simulink model "Rail_MonMeUn"  (R2016b)
settings: configuration reference "CodeGenConfigSet" (kept outside this file)
values from neighbouring files (symbols this model uses):
  Rail_dvolMeUnMonSetMin_C = Calibration.Parameter    [init_Rail_MonMeUn.m]
  Rail_dvolMeUnOvrRun_CUR = Calibration.Parameter    [init_Rail_MonMeUn.m]
  Rail_dvolMeUnOvrRun_CURX = Calibration.Parameter    [init_Rail_MonMeUn.m]
  Rail_dvolMonHPUnTolc_CUR = Calibration.Parameter    [init_Rail_MonMeUn.m]
  Rail_dvolMonHPUnTolc_CURX = Calibration.Parameter    [init_Rail_MonMeUn.m]
  Rail_dvolMonIdlMax_C = Calibration.Parameter    [init_Rail_MonMeUn.m]
  Rail_dvolMonLeakTolc_CUR = Calibration.Parameter    [init_Rail_MonMeUn.m]
  Rail_dvolMonLeakTolc_CURX = Calibration.Parameter    [init_Rail_MonMeUn.m]
  Rail_nMonIdlMax_C = Calibration.Parameter    [init_Rail_MonMeUn.m]
  Rail_pMeUnDvtMax_CUR = Calibration.Parameter    [init_Rail_MonMeUn.m]
  Rail_pMeUnDvtMax_CURX = Calibration.Parameter    [init_Rail_MonMeUn.m]
  Rail_pMeUnDvtMin2_CUR = Calibration.Parameter    [init_Rail_MonMeUn.m]
  Rail_pMeUnDvtMin2_CURX = Calibration.Parameter    [init_Rail_MonMeUn.m]
  Rail_pMeUnDvtMin_CUR = Calibration.Parameter    [init_Rail_MonMeUn.m]
  Rail_pMeUnDvtMin_CURX = Calibration.Parameter    [init_Rail_MonMeUn.m]
  Rail_pMeUnFltMin_CUR = Calibration.Parameter    [init_Rail_MonMeUn.m]
  Rail_pMeUnFltMin_CURX = Calibration.Parameter    [init_Rail_MonMeUn.m]
  Rail_pMeUnMonFltMax2_C = Calibration.Parameter    [init_Rail_MonMeUn.m]
  Rail_pMeUnMonFltMax_C = Calibration.Parameter    [init_Rail_MonMeUn.m]
  Rail_pMonDvtMax_C = Calibration.Parameter    [init_Rail_MonMeUn.m]
  Rail_qMeUnMonLoIdl_C = Calibration.Parameter    [init_Rail_MonMeUn.m]
  Rail_qMonUnBalMax_C = Calibration.Parameter    [init_Rail_MonMeUn.m]
  Rail_stMeUnMonRls_C = Calibration.Parameter    [init_Rail_MonMeUn.m]
  Rail_tiMeUn0Deb_C = Calibration.Parameter    [init_Rail_MonMeUn.m]
  Rail_tiMeUn10Deb_C = Calibration.Parameter    [init_Rail_MonMeUn.m]
  Rail_tiMeUn22Deb_C = Calibration.Parameter    [init_Rail_MonMeUn.m]
  Rail_tiMeUn2Deb_C = Calibration.Parameter    [init_Rail_MonMeUn.m]
  Rail_tiMeUn3Deb_C = Calibration.Parameter    [init_Rail_MonMeUn.m]
  Rail_tiMeUn42Deb_C = Calibration.Parameter    [init_Rail_MonMeUn.m]
  Rail_tiMeUn4Deb_C = Calibration.Parameter    [init_Rail_MonMeUn.m]
  Rail_tiMeUn7Deb_C = Calibration.Parameter    [init_Rail_MonMeUn.m]
  Rail_tiMeUn8Deb_C = Calibration.Parameter    [init_Rail_MonMeUn.m]
  Rail_tMeUnMonLoIdl_C = Calibration.Parameter    [init_Rail_MonMeUn.m]
undefined symbols (not defined in the file or in its folder): Rail_MonMeUn_DT, RailCtl_State_conv
libraries: CXLib x27, simulink x18
settings Model: Creator=lenovo  LastModifiedBy=liutao
settings ConfigSetRef: SourceLocation=Base Workspace

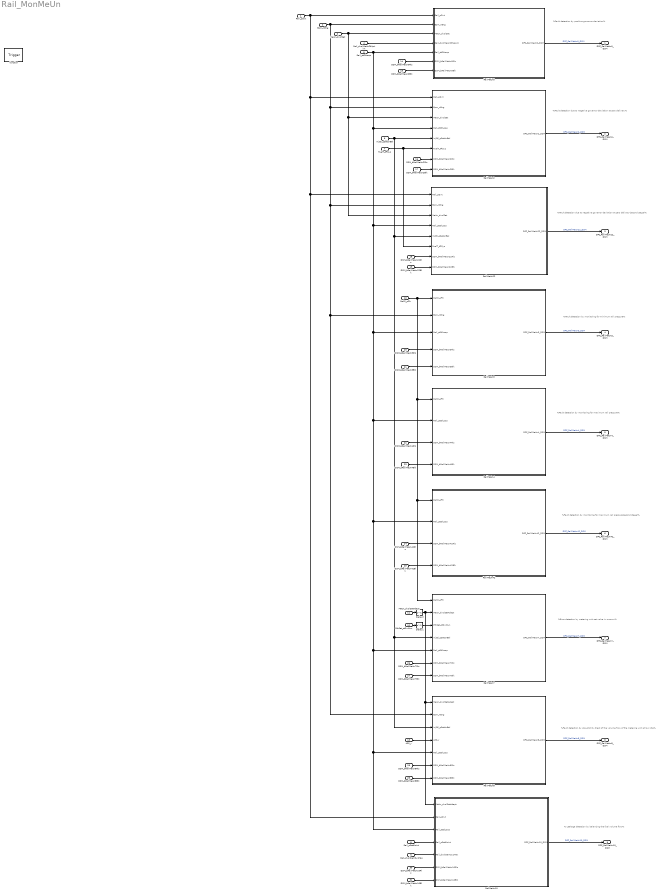
== system Rail_MonMeUn ==
  note: % Leakage detection by balancing the fuel volume flow%
  note: %Fault detection by plausibility check of the volume flow of the metering unit at low idle%
  note: %Error detection by metering unit set value in overrun%
  note: %Fault detection by monitoring for maximum rail pressure(second stage)%
  note: %Fault detection by monitoring for maximum rail pressure%
  note: %Fault detection by monitoring for minimum rail pressure%
  note: %Fault detection due to negative governor deviation at zero delivery(second stage)%
  note: %Fault detection due to negative governor deviation at zero delivery%
  note: %Fault detection by positive governor deviation%
  Rail_pDvt : Inport  Tag=bar  Description=Governor deviation of the rail pressure governor  OutMin=-2500  OutMax=2500  OutDataTypeStr=RailPressure_bar
  Epm_nEng : Inport  Tag=rpm  Description=Engine speed  Port=2  OutMin=0  OutMax=6000  OutDataTypeStr=EngSpeed_rpm
  MeUn_dvolSet : Inport  Tag=mm^3/s  Description=Setpoint value (volume flow) of rail pressure governing  Port=3  OutMin=-327670  OutMax=327670  OutDataTypeStr=FuelVol_mm3_s
  Rail_dvolMeUnCtlUpLim : Inport  Tag=mm^3/s  Description=Upper actuator value limit for pressure governing by metering unit  Port=4  OutMin=0  OutMax=327670  OutDataTypeStr=FuelVol_mm3_s
  Rail_stCtlLoop : Inport  Description=State of the rail pressure governor control  Port=5  OutDataTypeStr=Enum: RailCtl_State_conv
  InjCtl_qSetUnBal : Inport  Tag=mg/hub  Description=Current injection quantity  Port=6  OutMin=-319  OutMax=319  OutDataTypeStr=FuelMass_mg_hub
  FuelT_tFlSys : Inport  Tag=deg  Description=Fuel system temperature  Port=7  OutMin=-50  OutMax=200  OutDataTypeStr=Temp_deg
  Rail_pSetPoint : Inport  Tag=bar  Description=Rail pressure setpoint  Port=8  OutMin=-2500  OutMax=2500  OutDataTypeStr=RailPressure_bar
  Rail_dvolDemSysMax : Inport  Tag=mm^3/s  Description=Volume flow requested overall for a maximum tolerated injection system  Port=9  OutMin=-327680  OutMax=327670  OutDataTypeStr=FuelVol_mm3_s
  RailP_pFlt : Inport  Tag=bar  Description=Maximum rail pressure of the last 10 sampling cycle  Port=10  OutMin=0  OutMax=2500  OutDataTypeStr=RailPressure_bar
  MeUn_dvolSetAdapt : Inport  Tag=mm^3/s  Description=Correction value of the adaption of the metering unit  Port=11  OutMin=-327680  OutMax=327670  OutDataTypeStr=FuelVol_mm3_s
  PthSet_stOvrRun : Inport  Description=State of overrun detection (0: No overrun; 1: overrun)  Port=12  OutMin=0  OutMax=1  OutDataTypeStr=boolean
  APP_r : Inport  Tag=%  Description=Acceleration pedal sensor 1 value after fault handling  Port=13  OutMin=0  OutMax=100  OutDataTypeStr=Accpedal_rate
  DSM_bRailMeUn0Rls : Inport  Description=state of FId_RailMeUn0Rls  Port=14  OutMin=0  OutMax=1  OutDataTypeStr=boolean
  DSM_bRailMeUn0Blk : Inport  Description=state of FId_RailMeUn0Blk  Port=15  OutMin=0  OutMax=1  OutDataTypeStr=boolean
  DSM_bRailMeUn2Rls : Inport  Description=state of FId_RailMeUn2Rls  Port=16  OutMin=0  OutMax=1  OutDataTypeStr=boolean
  DSM_bRailMeUn2Blk : Inport  Description=state of FId_RailMeUn2Blk  Port=17  OutMin=0  OutMax=1  OutDataTypeStr=boolean
  DSM_bRailMeUn22Rls : Inport  Description=state of FId_RailMeUn22Rls  Port=18  OutMin=0  OutMax=1  OutDataTypeStr=boolean
  DSM_bRailMeUn22Blk : Inport  Description=state of FId_RailMeUn22Blk  Port=19  OutMin=0  OutMax=1  OutDataTypeStr=boolean
  DSM_bRailMeUn3Rls : Inport  Description=state of FId_RailMeUn3Rls  Port=20  OutMin=0  OutMax=1  OutDataTypeStr=boolean
  DSM_bRailMeUn3Blk : Inport  Description=state of FId_RailMeUn3Blk  Port=21  OutMin=0  OutMax=1  OutDataTypeStr=boolean
  DSM_bRailMeUn4Rls : Inport  Description=state of FId_RailMeUn4Rls  Port=22  OutMin=0  OutMax=1  OutDataTypeStr=boolean
  DSM_bRailMeUn4Blk : Inport  Description=state of FId_RailMeUn4Blk  Port=23  OutMin=0  OutMax=1  OutDataTypeStr=boolean
  DSM_bRailMeUn42Rls : Inport  Description=state of FId_RailMeUn42Rls  Port=24  OutMin=0  OutMax=1  OutDataTypeStr=boolean
  DSM_bRailMeUn42Blk : Inport  Description=state of FId_RailMeUn42Blk  Port=25  OutMin=0  OutMax=1  OutDataTypeStr=boolean
  DSM_bRailMeUn7Rls : Inport  Description=state of FId_RailMeUn7Rls  Port=26  OutMin=0  OutMax=1  OutDataTypeStr=boolean
  DSM_bRailMeUn7Blk : Inport  Description=state of FId_RailMeUn7Blk  Port=27  OutMin=0  OutMax=1  OutDataTypeStr=boolean
  DSM_bRailMeUn8Rls : Inport  Description=state of FId_RailMeUn8Rls  Port=28  OutMin=0  OutMax=1  OutDataTypeStr=boolean
  DSM_bRailMeUn8Blk : Inport  Description=state of FId_RailMeUn8Blk  Port=29  OutMin=0  OutMax=1  OutDataTypeStr=boolean
  DSM_bRailMeUn10Rls : Inport  Description=state of FId_RailMeUn10Rls  Port=30  OutMin=0  OutMax=1  OutDataTypeStr=boolean
  DSM_bRailMeUn10Blk : Inport  Description=state of FId_RailMeUn10Blk  Port=31  OutMin=0  OutMax=1  OutDataTypeStr=boolean
  function : TriggerPort  TriggerType=function-call  VariantControl=Variant
  Delay1 : Delay  DelayLength=1  InitialCondition=0
  Delay2 : Delay  DelayLength=1  InitialCondition=0
  RailMeUn0 : Subsystem
  RailMeUn10 : Subsystem
  RailMeUn2 : Subsystem
  RailMeUn22 : Subsystem
  RailMeUn3 : Subsystem
  RailMeUn4 : Subsystem
  RailMeUn42 : Subsystem
  RailMeUn7 : Subsystem
  RailMeUn8 : Subsystem
  DFC_RailMeUn0_DSM : Outport  Description=state of DFC_RailMeUn0  OutMin=0  OutMax=1  OutDataTypeStr=boolean
  DFC_RailMeUn2_DSM : Outport  Description=state of DFC_RailMeUn2  Port=2  OutMin=0  OutMax=1  OutDataTypeStr=boolean
  DFC_RailMeUn22_DSM : Outport  Description=state of DFC_RailMeUn22  Port=3  OutMin=0  OutMax=1  OutDataTypeStr=boolean
  DFC_RailMeUn3_DSM : Outport  Description=state of DFC_RailMeUn3  Port=4  OutMin=0  OutMax=1  OutDataTypeStr=boolean
  DFC_RailMeUn4_DSM : Outport  Description=state of DFC_RailMeUn4  Port=5  OutMin=0  OutMax=1  OutDataTypeStr=boolean
  DFC_RailMeUn42_DSM : Outport  Description=state of DFC_RailMeUn42  Port=6  OutMin=0  OutMax=1  OutDataTypeStr=boolean
  DFC_RailMeUn7_DSM : Outport  Description=state of DFC_RailMeUn7  Port=7  OutMin=0  OutMax=1  OutDataTypeStr=boolean
  DFC_RailMeUn8_DSM : Outport  Description=state of DFC_RailMeUn8  Port=8  OutMin=0  OutMax=1  OutDataTypeStr=boolean
  DFC_RailMeUn10_DSM : Outport  Description=state of DFC_RailMeUn10  Port=9  OutMin=0  OutMax=1  OutDataTypeStr=boolean
  wires:
  RailMeUn0/1(DFC_RailMeUn0_DSM) -> DFC_RailMeUn0_DSM/1  "DFC_RailMeUn0_DSM"
  RailMeUn2/1(DFC_RailMeUn2_DSM) -> DFC_RailMeUn2_DSM/1  "DFC_RailMeUn2_DSM"
  RailMeUn22/1(DFC_RailMeUn22_DSM) -> DFC_RailMeUn22_DSM/1  "DFC_RailMeUn22_DSM"
  RailMeUn3/1(DFC_RailMeUn3_DSM) -> DFC_RailMeUn3_DSM/1  "DFC_RailMeUn3_DSM"
  RailMeUn4/1(DFC_RailMeUn4_DSM) -> DFC_RailMeUn4_DSM/1  "DFC_RailMeUn4_DSM"
  RailMeUn42/1(DFC_RailMeUn42_DSM) -> DFC_RailMeUn42_DSM/1  "DFC_RailMeUn42_DSM"
  RailMeUn7/1(DFC_RailMeUn7_DSM) -> DFC_RailMeUn7_DSM/1  "DFC_RailMeUn7_DSM"
  RailMeUn8/1(DFC_RailMeUn8_DSM) -> DFC_RailMeUn8_DSM/1  "DFC_RailMeUn8_DSM"
  RailMeUn10/1(DFC_RailMeUn10_DSM) -> DFC_RailMeUn10_DSM/1  "DFC_RailMeUn10_DSM"
  Rail_stCtlLoop/1 -> RailMeUn10/3(Rail_stCtlLoop), RailMeUn8/5(Rail_stCtlLoop), RailMeUn7/5(Rail_stCtlLoop), RailMeUn42/2(Rail_stCtlLoop), RailMeUn4/2(Rail_stCtlLoop), RailMeUn3/3(Rail_stCtlLoop), RailMeUn22/4(Rail_stCtlLoop), RailMeUn2/4(Rail_stCtlLoop), RailMeUn0/5(Rail_stCtlLoop)
  Rail_dvolDemSysMax/1 -> RailMeUn10/5(Rail_dvolDemSysMax)
  Rail_pSetPoint/1 -> RailMeUn10/4(Rail_pSetPoint)
  APP_r/1 -> RailMeUn8/4(APP_r)
  PthSet_stOvrRun/1 -> Delay1/1
  MeUn_dvolSetAdapt/1 -> Delay2/1
  RailP_pFlt/1 -> RailMeUn7/1(RailP_pFlt), RailMeUn42/1(RailP_pFlt), RailMeUn4/1(RailP_pFlt), RailMeUn3/1(RailP_pFlt)
  FuelT_tFlSys/1 -> RailMeUn2/6(FuelT_tFlSys), RailMeUn22/6(FuelT_tFlSys)
  InjCtl_qSetUnBal/1 -> RailMeUn2/5(InjCtl_qSetUnBal), RailMeUn8/3(InjCtl_qSetUnBal), RailMeUn7/4(InjCtl_qSetUnBal), RailMeUn22/5(InjCtl_qSetUnBal)
  Rail_dvolMeUnCtlUpLim/1 -> RailMeUn0/4(Rail_dvolMeUnCtlUpLim)
  MeUn_dvolSet/1 -> RailMeUn0/3(MeUn_dvolSet), RailMeUn22/3(MeUn_dvolSet), RailMeUn2/3(MeUn_dvolSet)
  Rail_pDvt/1 -> RailMeUn10/2(Rail_pDvt), RailMeUn22/1(Rail_pDvt), RailMeUn2/1(Rail_pDvt), RailMeUn0/1(Rail_pDvt)
  Epm_nEng/1 -> RailMeUn8/2(Epm_nEng), RailMeUn3/2(Epm_nEng), RailMeUn22/2(Epm_nEng), RailMeUn2/2(Epm_nEng), RailMeUn0/2(Epm_nEng)
  DSM_bRailMeUn0Rls/1 -> RailMeUn0/6(DSM_bRailMeUn0Rls)
  DSM_bRailMeUn0Blk/1 -> RailMeUn0/7(DSM_bRailMeUn0Blk)
  DSM_bRailMeUn2Blk/1 -> RailMeUn2/8(DSM_bRailMeUn2Blk)
  DSM_bRailMeUn2Rls/1 -> RailMeUn2/7(DSM_bRailMeUn2Rls)
  DSM_bRailMeUn22Rls/1 -> RailMeUn22/7(DSM_bRailMeUn22Rls)
  DSM_bRailMeUn22Blk/1 -> RailMeUn22/8(DSM_bRailMeUn22Blk)
  DSM_bRailMeUn3Rls/1 -> RailMeUn3/4(DSM_bRailMeUn3Rls)
  DSM_bRailMeUn3Blk/1 -> RailMeUn3/5(DSM_bRailMeUn3Blk)
  DSM_bRailMeUn4Rls/1 -> RailMeUn4/3(DSM_bRailMeUn4Rls)
  DSM_bRailMeUn4Blk/1 -> RailMeUn4/4(DSM_bRailMeUn4Blk)
  DSM_bRailMeUn42Rls/1 -> RailMeUn42/3(DSM_bRailMeUn42Rls)
  DSM_bRailMeUn42Blk/1 -> RailMeUn42/4(DSM_bRailMeUn42Blk)
  DSM_bRailMeUn7Rls/1 -> RailMeUn7/6(DSM_bRailMeUn7Rls)
  DSM_bRailMeUn7Blk/1 -> RailMeUn7/7(DSM_bRailMeUn7Blk)
  DSM_bRailMeUn8Rls/1 -> RailMeUn8/6(DSM_bRailMeUn8Rls)
  DSM_bRailMeUn8Blk/1 -> RailMeUn8/7(DSM_bRailMeUn8Blk)
  DSM_bRailMeUn10Rls/1 -> RailMeUn10/6(DSM_bRailMeUn10Rls)
  DSM_bRailMeUn10Blk/1 -> RailMeUn10/7(DSM_bRailMeUn10Blk)
  Delay1/1 -> RailMeUn7/3(PthSet_stOvrRun)
  Delay2/1 -> RailMeUn10/1(MeUn_dvolSetAdapt), RailMeUn8/1(MeUn_dvolSetAdapt), RailMeUn7/2(MeUn_dvolSetAdapt)

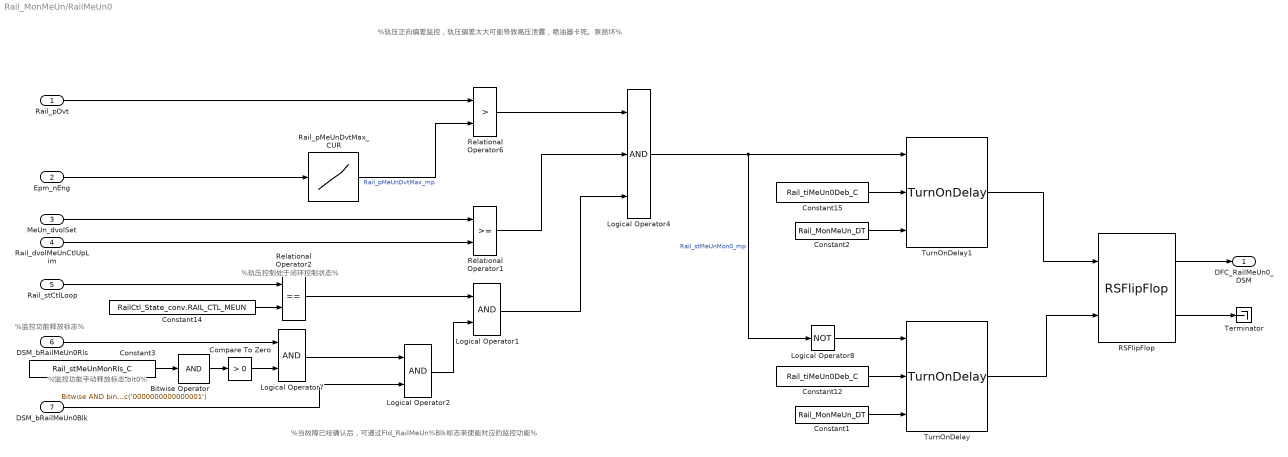
== system Rail_MonMeUn/RailMeUn0 ==
  note: %当故障已经确认后，可通过FId_RailMeUn%Blk标志来使能对应的监控功能%
  note: %监控功能释放标志%
  note: %轨压控制处于闭环控制状态%
  note: %轨压正向偏差监控，轨压偏差太大可能导致高压泄露，喷油器卡死。泵损坏%
  note: %监控功能手动释放标志,bit0%
  Rail_pDvt : Inport
  Epm_nEng : Inport  Port=2
  MeUn_dvolSet : Inport  Port=3
  Rail_dvolMeUnCtlUpLim : Inport  Port=4
  Rail_stCtlLoop : Inport  Port=5
  DSM_bRailMeUn0Rls : Inport  Description=state of FId_RailMeUn0Rls  Port=6  OutMin=0  OutMax=1  OutDataTypeStr=boolean
  DSM_bRailMeUn0Blk : Inport  Description=state of FId_RailMeUn0Blk  Port=7  OutMin=0  OutMax=1  OutDataTypeStr=boolean
  Bitwise Operator : simulink/Logic and Bit Operations/Bitwise Operator  logicop=AND  UseBitMask=on  BitMask=bin2dec('0000000000000001')  BitMaskRealWorld=Stored Integer
  Compare To Zero : simulink/Logic and Bit Operations/Compare To Zero  relop=>  OutDataTypeStr=boolean
  Constant1 : Constant  Value=Rail_MonMeUn_DT  OutDataTypeStr=Inherit: Inherit via back propagation
  Constant12 : Constant  Value=Rail_tiMeUn0Deb_C
  Constant14 : Constant  Value=RailCtl_State_conv.RAIL_CTL_MEUN
  Constant15 : Constant  Value=Rail_tiMeUn0Deb_C
  Constant2 : Constant  Value=Rail_MonMeUn_DT  OutDataTypeStr=Inherit: Inherit via back propagation
  Constant3 : Constant  Value=Rail_stMeUnMonRls_C
  Logical Operator1 : Logic  AllPortsSameDT=off  OutDataTypeStr=boolean
  Logical Operator2 : Logic  AllPortsSameDT=off  OutDataTypeStr=boolean
  Logical Operator4 : Logic  Inputs=3  AllPortsSameDT=off  OutDataTypeStr=boolean
  Logical Operator7 : Logic  OutDataTypeStr=boolean
  Logical Operator8 : Logic  Operator=NOT  AllPortsSameDT=off  OutDataTypeStr=boolean
  RSFlipFlop : CXLib/RSFlipFlop
  Rail_pMeUnDvtMax_CUR : Lookup_n-D  NumberOfTableDimensions=1  BreakpointsForDimension1=Rail_pMeUnDvtMax_CURX  IndexSearchMethod=Linear search  Table=Rail_pMeUnDvtMax_CUR  ExtrapMethod=Clip  InternalRulePriority=Speed  OutDataTypeStr=Inherit: Inherit via back propagation  RndMeth=Simplest  SaturateOnIntegerOverflow=on
  Relational Operator1 : RelationalOperator  OutDataTypeStr=boolean  RndMeth=Nearest  InputSameDT=on
  Relational Operator2 : RelationalOperator  Operator===  OutDataTypeStr=boolean  RndMeth=Nearest  InputSameDT=on
  Relational Operator6 : RelationalOperator  Operator=>  OutDataTypeStr=boolean  RndMeth=Nearest  InputSameDT=on
  Terminator : Terminator
  TurnOnDelay : CXLib/TurnOnDelay
  TurnOnDelay1 : CXLib/TurnOnDelay
  DFC_RailMeUn0_DSM : Outport  Description=state of DFC_RailMeUn0  OutMin=0  OutMax=1  OutDataTypeStr=boolean
  wires:
  Constant2/1 -> TurnOnDelay1/3
  Constant1/1 -> TurnOnDelay/3
  TurnOnDelay1/1 -> RSFlipFlop/1
  TurnOnDelay/1 -> RSFlipFlop/2
  Constant12/1 -> TurnOnDelay/2
  Logical Operator8/1 -> TurnOnDelay/1
  Constant15/1 -> TurnOnDelay1/2
  Logical Operator7/1 -> Logical Operator2/1
  DSM_bRailMeUn0Rls/1 -> Logical Operator7/1
  Logical Operator4/1 -> Logical Operator8/1, TurnOnDelay1/1  "Rail_stMeUnMon0_mp"
  DSM_bRailMeUn0Blk/1 -> Logical Operator2/2
  Logical Operator2/1 -> Logical Operator1/2
  Relational Operator2/1 -> Logical Operator1/1
  Constant14/1 -> Relational Operator2/2
  Logical Operator1/1 -> Logical Operator4/3
  Rail_dvolMeUnCtlUpLim/1 -> Relational Operator1/2
  Relational Operator1/1 -> Logical Operator4/2
  Relational Operator6/1 -> Logical Operator4/1
  Rail_pMeUnDvtMax_CUR/1 -> Relational Operator6/2  "Rail_pMeUnDvtMax_mp"
  Rail_stCtlLoop/1 -> Relational Operator2/1
  MeUn_dvolSet/1 -> Relational Operator1/1
  Rail_pDvt/1 -> Relational Operator6/1
  Epm_nEng/1 -> Rail_pMeUnDvtMax_CUR/1
  RSFlipFlop/1 -> DFC_RailMeUn0_DSM/1
  RSFlipFlop/2 -> Terminator/1
  Bitwise Operator/1 -> Compare To Zero/1
  Constant3/1 -> Bitwise Operator/1
  Compare To Zero/1 -> Logical Operator7/2

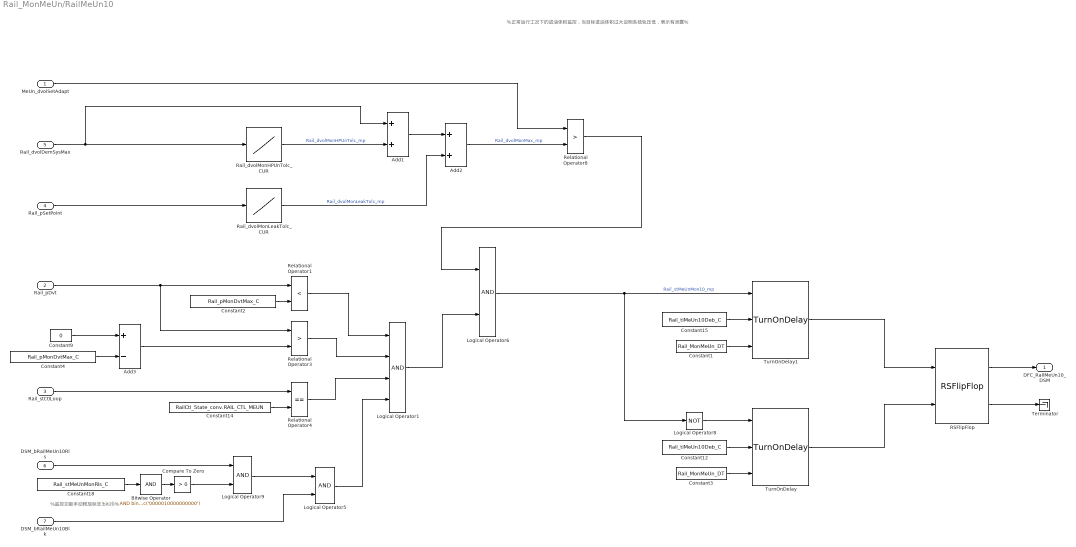
== system Rail_MonMeUn/RailMeUn10 ==
  note: %正常运行工况下的进油体积监控，当目标进油体积过大说明系统轨压低，表示有泄露%
  note: %监控功能手动释放标志,bit10%
  MeUn_dvolSetAdapt : Inport
  Rail_pDvt : Inport  Port=2
  Rail_stCtlLoop : Inport  Port=3
  Rail_pSetPoint : Inport  Port=4
  Rail_dvolDemSysMax : Inport  Port=5
  DSM_bRailMeUn10Rls : Inport  Description=state of FId_RailMeUn10Rls  Port=6  OutMin=0  OutMax=1  OutDataTypeStr=boolean
  DSM_bRailMeUn10Blk : Inport  Description=state of FId_RailMeUn10Blk  Port=7  OutMin=0  OutMax=1  OutDataTypeStr=boolean
  Add1 : Sum  InputSameDT=on
  Add2 : Sum  InputSameDT=on
  Add3 : Sum  Inputs=+-  InputSameDT=on
  Bitwise Operator : simulink/Logic and Bit Operations/Bitwise Operator  logicop=AND  UseBitMask=on  BitMask=bin2dec('0000010000000000')  BitMaskRealWorld=Stored Integer
  Compare To Zero : simulink/Logic and Bit Operations/Compare To Zero  relop=>  OutDataTypeStr=boolean
  Constant1 : Constant  Value=Rail_MonMeUn_DT  OutDataTypeStr=Inherit: Inherit via back propagation
  Constant12 : Constant  Value=Rail_tiMeUn10Deb_C
  Constant14 : Constant  Value=RailCtl_State_conv.RAIL_CTL_MEUN
  Constant15 : Constant  Value=Rail_tiMeUn10Deb_C
  Constant18 : Constant  Value=Rail_stMeUnMonRls_C
  Constant2 : Constant  Value=Rail_pMonDvtMax_C
  Constant3 : Constant  Value=Rail_MonMeUn_DT  OutDataTypeStr=Inherit: Inherit via back propagation
  Constant4 : Constant  Value=Rail_pMonDvtMax_C
  Constant9 : Constant  Value=0  OutDataTypeStr=Inherit: Inherit via back propagation
  Logical Operator1 : Logic  Inputs=4  AllPortsSameDT=off  OutDataTypeStr=boolean
  Logical Operator5 : Logic  AllPortsSameDT=off  OutDataTypeStr=boolean
  Logical Operator6 : Logic  AllPortsSameDT=off  OutDataTypeStr=boolean
  Logical Operator8 : Logic  Operator=NOT  AllPortsSameDT=off  OutDataTypeStr=boolean
  Logical Operator9 : Logic  AllPortsSameDT=off  OutDataTypeStr=boolean
  RSFlipFlop : CXLib/RSFlipFlop
  Rail_dvolMonHPUnTolc_CUR : Lookup_n-D  NumberOfTableDimensions=1  BreakpointsForDimension1=Rail_dvolMonHPUnTolc_CURX  IndexSearchMethod=Linear search  Table=Rail_dvolMonHPUnTolc_CUR  ExtrapMethod=Clip  InternalRulePriority=Speed  OutDataTypeStr=Inherit: Inherit via back propagation  RndMeth=Simplest  SaturateOnIntegerOverflow=on
  Rail_dvolMonLeakTolc_CUR : Lookup_n-D  NumberOfTableDimensions=1  BreakpointsForDimension1=Rail_dvolMonLeakTolc_CURX  IndexSearchMethod=Linear search  Table=Rail_dvolMonLeakTolc_CUR  ExtrapMethod=Clip  InternalRulePriority=Speed  OutDataTypeStr=Inherit: Inherit via back propagation  RndMeth=Simplest  SaturateOnIntegerOverflow=on
  Relational Operator1 : RelationalOperator  Operator=<  OutDataTypeStr=boolean  RndMeth=Nearest  InputSameDT=on
  Relational Operator3 : RelationalOperator  Operator=>  OutDataTypeStr=boolean  RndMeth=Nearest  InputSameDT=on
  Relational Operator4 : RelationalOperator  Operator===  OutDataTypeStr=boolean  RndMeth=Nearest  InputSameDT=on
  Relational Operator8 : RelationalOperator  Operator=>  OutDataTypeStr=boolean  RndMeth=Nearest  InputSameDT=on
  Terminator : Terminator
  TurnOnDelay : CXLib/TurnOnDelay
  TurnOnDelay1 : CXLib/TurnOnDelay
  DFC_RailMeUn10_DSM : Outport  Description=state of DFC_RailMeUn10  OutMin=0  OutMax=1  OutDataTypeStr=boolean
  wires:
  Constant1/1 -> TurnOnDelay1/3
  Constant3/1 -> TurnOnDelay/3
  Logical Operator8/1 -> TurnOnDelay/1
  TurnOnDelay1/1 -> RSFlipFlop/1
  TurnOnDelay/1 -> RSFlipFlop/2
  Constant12/1 -> TurnOnDelay/2
  Constant15/1 -> TurnOnDelay1/2
  Logical Operator6/1 -> TurnOnDelay1/1, Logical Operator8/1  "Rail_stMeUnMon10_mp"
  Relational Operator4/1 -> Logical Operator1/3
  Logical Operator5/1 -> Logical Operator1/4
  Relational Operator3/1 -> Logical Operator1/2
  Constant4/1 -> Add3/2
  Constant9/1 -> Add3/1
  Add3/1 -> Relational Operator3/2
  Relational Operator1/1 -> Logical Operator1/1
  Relational Operator8/1 -> Logical Operator6/1
  MeUn_dvolSetAdapt/1 -> Relational Operator8/1
  Add2/1 -> Relational Operator8/2  "Rail_dvolMonMax_mp"
  Add1/1 -> Add2/1
  Rail_dvolMonLeakTolc_CUR/1 -> Add2/2  "Rail_dvolMonLeakTolc_mp"
  Rail_dvolDemSysMax/1 -> Add1/1, Rail_dvolMonHPUnTolc_CUR/1
  Rail_pSetPoint/1 -> Rail_dvolMonLeakTolc_CUR/1
  Rail_dvolMonHPUnTolc_CUR/1 -> Add1/2  "Rail_dvolMonHPUnTolc_mp"
  Rail_pDvt/1 -> Relational Operator1/1, Relational Operator3/1
  Logical Operator1/1 -> Logical Operator6/2
  DSM_bRailMeUn10Blk/1 -> Logical Operator5/2
  Logical Operator9/1 -> Logical Operator5/1
  DSM_bRailMeUn10Rls/1 -> Logical Operator9/1
  Constant2/1 -> Relational Operator1/2
  Constant14/1 -> Relational Operator4/2
  Rail_stCtlLoop/1 -> Relational Operator4/1
  RSFlipFlop/1 -> DFC_RailMeUn10_DSM/1
  RSFlipFlop/2 -> Terminator/1
  Bitwise Operator/1 -> Compare To Zero/1
  Constant18/1 -> Bitwise Operator/1
  Compare To Zero/1 -> Logical Operator9/2

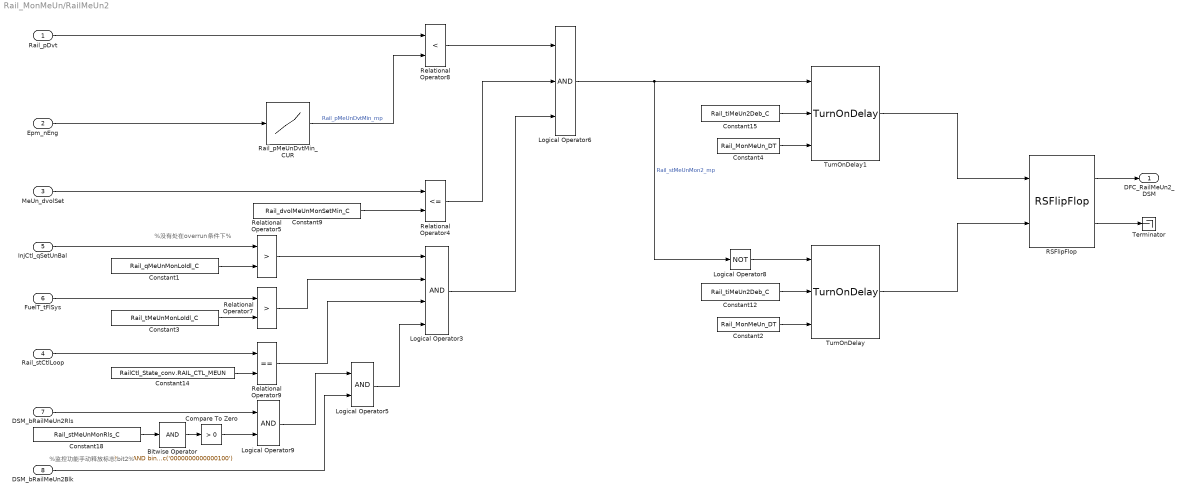
== system Rail_MonMeUn/RailMeUn2 ==
  note: %没有处在overrun条件下%
  note: %监控功能手动释放标志,bit2%
  Rail_pDvt : Inport
  Epm_nEng : Inport  Port=2
  MeUn_dvolSet : Inport  Port=3
  Rail_stCtlLoop : Inport  Port=4
  InjCtl_qSetUnBal : Inport  Port=5
  FuelT_tFlSys : Inport  Port=6
  DSM_bRailMeUn2Rls : Inport  Description=state of FId_RailMeUn2Rls  Port=7  OutMin=0  OutMax=1  OutDataTypeStr=boolean
  DSM_bRailMeUn2Blk : Inport  Description=state of FId_RailMeUn2Blk  Port=8  OutMin=0  OutMax=1  OutDataTypeStr=boolean
  Bitwise Operator : simulink/Logic and Bit Operations/Bitwise Operator  logicop=AND  UseBitMask=on  BitMask=bin2dec('0000000000000100')  BitMaskRealWorld=Stored Integer
  Compare To Zero : simulink/Logic and Bit Operations/Compare To Zero  relop=>  OutDataTypeStr=boolean
  Constant1 : Constant  Value=Rail_qMeUnMonLoIdl_C
  Constant12 : Constant  Value=Rail_tiMeUn2Deb_C
  Constant14 : Constant  Value=RailCtl_State_conv.RAIL_CTL_MEUN
  Constant15 : Constant  Value=Rail_tiMeUn2Deb_C
  Constant18 : Constant  Value=Rail_stMeUnMonRls_C
  Constant2 : Constant  Value=Rail_MonMeUn_DT  OutDataTypeStr=Inherit: Inherit via back propagation
  Constant3 : Constant  Value=Rail_tMeUnMonLoIdl_C
  Constant4 : Constant  Value=Rail_MonMeUn_DT  OutDataTypeStr=Inherit: Inherit via back propagation
  Constant9 : Constant  Value=Rail_dvolMeUnMonSetMin_C
  Logical Operator3 : Logic  Inputs=4  AllPortsSameDT=off  OutDataTypeStr=boolean
  Logical Operator5 : Logic  AllPortsSameDT=off  OutDataTypeStr=boolean
  Logical Operator6 : Logic  Inputs=3  AllPortsSameDT=off  OutDataTypeStr=boolean
  Logical Operator8 : Logic  Operator=NOT  AllPortsSameDT=off  OutDataTypeStr=boolean
  Logical Operator9 : Logic  AllPortsSameDT=off  OutDataTypeStr=boolean
  RSFlipFlop : CXLib/RSFlipFlop
  Rail_pMeUnDvtMin_CUR : Lookup_n-D  NumberOfTableDimensions=1  BreakpointsForDimension1=Rail_pMeUnDvtMin_CURX  IndexSearchMethod=Linear search  Table=Rail_pMeUnDvtMin_CUR  ExtrapMethod=Clip  InternalRulePriority=Speed  OutDataTypeStr=Inherit: Inherit via back propagation  RndMeth=Simplest  SaturateOnIntegerOverflow=on
  Relational Operator4 : RelationalOperator  Operator=<=  OutDataTypeStr=boolean  RndMeth=Nearest  InputSameDT=on
  Relational Operator5 : RelationalOperator  Operator=>  OutDataTypeStr=boolean  RndMeth=Nearest  InputSameDT=on
  Relational Operator7 : RelationalOperator  Operator=>  OutDataTypeStr=boolean  RndMeth=Nearest  InputSameDT=on
  Relational Operator8 : RelationalOperator  Operator=<  OutDataTypeStr=boolean  RndMeth=Nearest  InputSameDT=on
  Relational Operator9 : RelationalOperator  Operator===  OutDataTypeStr=boolean  RndMeth=Nearest  InputSameDT=on
  Terminator : Terminator
  TurnOnDelay : CXLib/TurnOnDelay
  TurnOnDelay1 : CXLib/TurnOnDelay
  DFC_RailMeUn2_DSM : Outport  Description=state of DFC_RailMeUn2  OutMin=0  OutMax=1  OutDataTypeStr=boolean
  wires:
  Constant4/1 -> TurnOnDelay1/3
  Constant2/1 -> TurnOnDelay/3
  TurnOnDelay1/1 -> RSFlipFlop/1
  TurnOnDelay/1 -> RSFlipFlop/2
  Constant12/1 -> TurnOnDelay/2
  Logical Operator8/1 -> TurnOnDelay/1
  Constant15/1 -> TurnOnDelay1/2
  Logical Operator6/1 -> TurnOnDelay1/1, Logical Operator8/1  "Rail_stMeUnMon2_mp"
  DSM_bRailMeUn2Blk/1 -> Logical Operator5/2
  Logical Operator9/1 -> Logical Operator5/1
  DSM_bRailMeUn2Rls/1 -> Logical Operator9/1
  Logical Operator5/1 -> Logical Operator3/4
  Relational Operator9/1 -> Logical Operator3/3
  Constant14/1 -> Relational Operator9/2
  Relational Operator7/1 -> Logical Operator3/2
  FuelT_tFlSys/1 -> Relational Operator7/1
  Constant1/1 -> Relational Operator5/2
  InjCtl_qSetUnBal/1 -> Relational Operator5/1
  Constant9/1 -> Relational Operator4/2
  Constant3/1 -> Relational Operator7/2
  Relational Operator5/1 -> Logical Operator3/1
  Logical Operator3/1 -> Logical Operator6/3
  Relational Operator4/1 -> Logical Operator6/2
  Relational Operator8/1 -> Logical Operator6/1
  Rail_pMeUnDvtMin_CUR/1 -> Relational Operator8/2  "Rail_pMeUnDvtMin_mp"
  Epm_nEng/1 -> Rail_pMeUnDvtMin_CUR/1
  MeUn_dvolSet/1 -> Relational Operator4/1
  Rail_pDvt/1 -> Relational Operator8/1
  Rail_stCtlLoop/1 -> Relational Operator9/1
  RSFlipFlop/1 -> DFC_RailMeUn2_DSM/1
  RSFlipFlop/2 -> Terminator/1
  Bitwise Operator/1 -> Compare To Zero/1
  Constant18/1 -> Bitwise Operator/1
  Compare To Zero/1 -> Logical Operator9/2

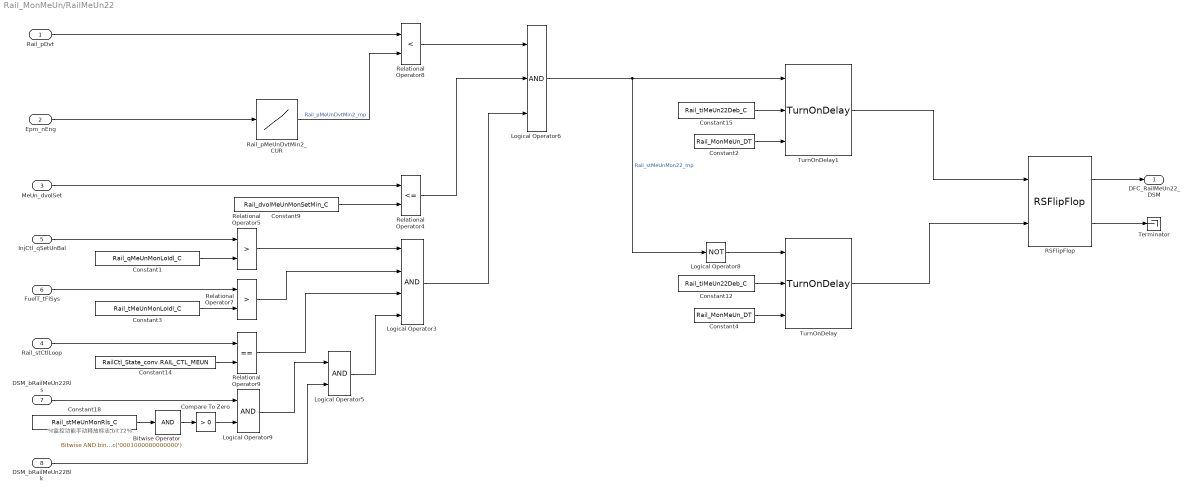
== system Rail_MonMeUn/RailMeUn22 ==
  note: %监控功能手动释放标志,bit12%
  Rail_pDvt : Inport
  Epm_nEng : Inport  Port=2
  MeUn_dvolSet : Inport  Port=3
  Rail_stCtlLoop : Inport  Port=4
  InjCtl_qSetUnBal : Inport  Port=5
  FuelT_tFlSys : Inport  Port=6
  DSM_bRailMeUn22Rls : Inport  Description=state of FId_RailMeUn22Rls  Port=7  OutMin=0  OutMax=1  OutDataTypeStr=boolean
  DSM_bRailMeUn22Blk : Inport  Description=state of FId_RailMeUn22Blk  Port=8  OutMin=0  OutMax=1  OutDataTypeStr=boolean
  Bitwise Operator : simulink/Logic and Bit Operations/Bitwise Operator  logicop=AND  UseBitMask=on  BitMask=bin2dec('0001000000000000')  BitMaskRealWorld=Stored Integer
  Compare To Zero : simulink/Logic and Bit Operations/Compare To Zero  relop=>  OutDataTypeStr=boolean
  Constant1 : Constant  Value=Rail_qMeUnMonLoIdl_C
  Constant12 : Constant  Value=Rail_tiMeUn22Deb_C
  Constant14 : Constant  Value=RailCtl_State_conv.RAIL_CTL_MEUN
  Constant15 : Constant  Value=Rail_tiMeUn22Deb_C
  Constant18 : Constant  Value=Rail_stMeUnMonRls_C
  Constant2 : Constant  Value=Rail_MonMeUn_DT  OutDataTypeStr=Inherit: Inherit via back propagation
  Constant3 : Constant  Value=Rail_tMeUnMonLoIdl_C
  Constant4 : Constant  Value=Rail_MonMeUn_DT  OutDataTypeStr=Inherit: Inherit via back propagation
  Constant9 : Constant  Value=Rail_dvolMeUnMonSetMin_C
  Logical Operator3 : Logic  Inputs=4  AllPortsSameDT=off  OutDataTypeStr=boolean
  Logical Operator5 : Logic  AllPortsSameDT=off  OutDataTypeStr=boolean
  Logical Operator6 : Logic  Inputs=3  AllPortsSameDT=off  OutDataTypeStr=boolean
  Logical Operator8 : Logic  Operator=NOT  AllPortsSameDT=off  OutDataTypeStr=boolean
  Logical Operator9 : Logic  AllPortsSameDT=off  OutDataTypeStr=boolean
  RSFlipFlop : CXLib/RSFlipFlop
  Rail_pMeUnDvtMin2_CUR : Lookup_n-D  NumberOfTableDimensions=1  BreakpointsForDimension1=Rail_pMeUnDvtMin2_CURX  IndexSearchMethod=Linear search  Table=Rail_pMeUnDvtMin2_CUR  ExtrapMethod=Clip  InternalRulePriority=Speed  OutDataTypeStr=Inherit: Inherit via back propagation  RndMeth=Simplest  SaturateOnIntegerOverflow=on
  Relational Operator4 : RelationalOperator  Operator=<=  OutDataTypeStr=boolean  RndMeth=Nearest  InputSameDT=on
  Relational Operator5 : RelationalOperator  Operator=>  OutDataTypeStr=boolean  RndMeth=Nearest  InputSameDT=on
  Relational Operator7 : RelationalOperator  Operator=>  OutDataTypeStr=boolean  RndMeth=Nearest  InputSameDT=on
  Relational Operator8 : RelationalOperator  Operator=<  OutDataTypeStr=boolean  RndMeth=Nearest  InputSameDT=on
  Relational Operator9 : RelationalOperator  Operator===  OutDataTypeStr=boolean  RndMeth=Nearest  InputSameDT=on
  Terminator : Terminator
  TurnOnDelay : CXLib/TurnOnDelay
  TurnOnDelay1 : CXLib/TurnOnDelay
  DFC_RailMeUn22_DSM : Outport  Description=state of DFC_RailMeUn22  OutMin=0  OutMax=1  OutDataTypeStr=boolean
  wires:
  Constant2/1 -> TurnOnDelay1/3
  Constant4/1 -> TurnOnDelay/3
  TurnOnDelay1/1 -> RSFlipFlop/1
  TurnOnDelay/1 -> RSFlipFlop/2
  Constant12/1 -> TurnOnDelay/2
  Logical Operator8/1 -> TurnOnDelay/1
  Constant15/1 -> TurnOnDelay1/2
  Logical Operator6/1 -> TurnOnDelay1/1, Logical Operator8/1  "Rail_stMeUnMon22_mp"
  Logical Operator3/1 -> Logical Operator6/3
  Relational Operator4/1 -> Logical Operator6/2
  Relational Operator8/1 -> Logical Operator6/1
  Rail_stCtlLoop/1 -> Relational Operator9/1
  Rail_pDvt/1 -> Relational Operator8/1
  MeUn_dvolSet/1 -> Relational Operator4/1
  Epm_nEng/1 -> Rail_pMeUnDvtMin2_CUR/1
  Rail_pMeUnDvtMin2_CUR/1 -> Relational Operator8/2  "Rail_pMeUnDvtMin2_mp"
  Relational Operator5/1 -> Logical Operator3/1
  Constant3/1 -> Relational Operator7/2
  Constant9/1 -> Relational Operator4/2
  InjCtl_qSetUnBal/1 -> Relational Operator5/1
  Constant1/1 -> Relational Operator5/2
  FuelT_tFlSys/1 -> Relational Operator7/1
  Relational Operator7/1 -> Logical Operator3/2
  Constant14/1 -> Relational Operator9/2
  Relational Operator9/1 -> Logical Operator3/3
  Logical Operator5/1 -> Logical Operator3/4
  DSM_bRailMeUn22Rls/1 -> Logical Operator9/1
  Logical Operator9/1 -> Logical Operator5/1
  DSM_bRailMeUn22Blk/1 -> Logical Operator5/2
  RSFlipFlop/1 -> DFC_RailMeUn22_DSM/1
  RSFlipFlop/2 -> Terminator/1
  Bitwise Operator/1 -> Compare To Zero/1
  Constant18/1 -> Bitwise Operator/1
  Compare To Zero/1 -> Logical Operator9/2

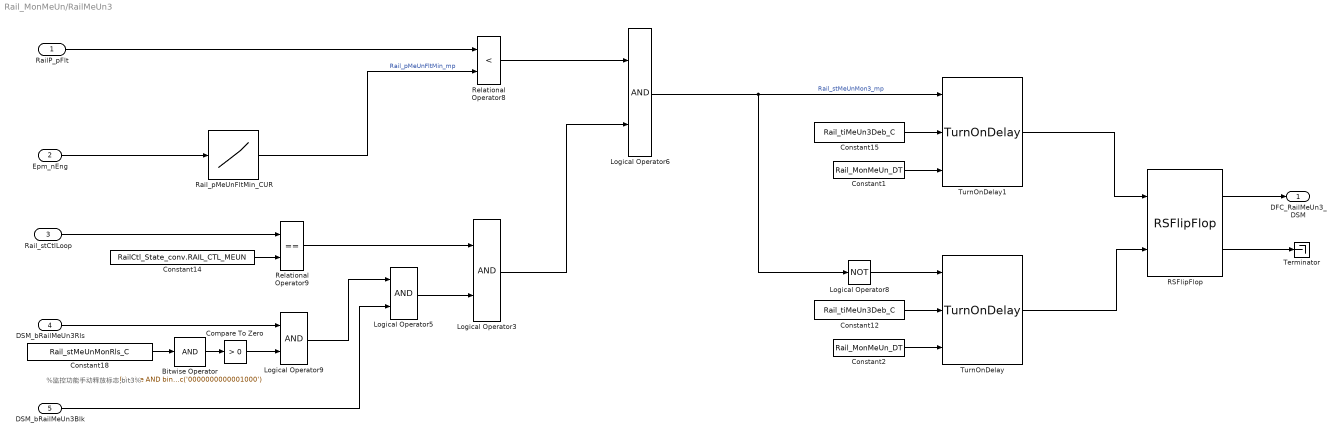
== system Rail_MonMeUn/RailMeUn3 ==
  note: %监控功能手动释放标志,bit3%
  RailP_pFlt : Inport
  Epm_nEng : Inport  Port=2
  Rail_stCtlLoop : Inport  Port=3
  DSM_bRailMeUn3Rls : Inport  Description=state of FId_RailMeUn3Rls  Port=4  OutMin=0  OutMax=1  OutDataTypeStr=boolean
  DSM_bRailMeUn3Blk : Inport  Description=state of FId_RailMeUn3Blk  Port=5  OutMin=0  OutMax=1  OutDataTypeStr=boolean
  Bitwise Operator : simulink/Logic and Bit Operations/Bitwise Operator  logicop=AND  UseBitMask=on  BitMask=bin2dec('0000000000001000')  BitMaskRealWorld=Stored Integer
  Compare To Zero : simulink/Logic and Bit Operations/Compare To Zero  relop=>  OutDataTypeStr=boolean
  Constant1 : Constant  Value=Rail_MonMeUn_DT  OutDataTypeStr=Inherit: Inherit via back propagation
  Constant12 : Constant  Value=Rail_tiMeUn3Deb_C
  Constant14 : Constant  Value=RailCtl_State_conv.RAIL_CTL_MEUN
  Constant15 : Constant  Value=Rail_tiMeUn3Deb_C
  Constant18 : Constant  Value=Rail_stMeUnMonRls_C
  Constant2 : Constant  Value=Rail_MonMeUn_DT  OutDataTypeStr=Inherit: Inherit via back propagation
  Logical Operator{3,5..6,9} (4 alike) : Logic  AllPortsSameDT=off  OutDataTypeStr=boolean
  Logical Operator8 : Logic  Operator=NOT  AllPortsSameDT=off  OutDataTypeStr=boolean
  RSFlipFlop : CXLib/RSFlipFlop
  Rail_pMeUnFltMin_CUR : Lookup_n-D  NumberOfTableDimensions=1  BreakpointsForDimension1=Rail_pMeUnFltMin_CURX  IndexSearchMethod=Linear search  Table=Rail_pMeUnFltMin_CUR  ExtrapMethod=Clip  InternalRulePriority=Speed  OutDataTypeStr=Inherit: Inherit via back propagation  RndMeth=Simplest  SaturateOnIntegerOverflow=on
  Relational Operator8 : RelationalOperator  Operator=<  OutDataTypeStr=boolean  RndMeth=Nearest  InputSameDT=on
  Relational Operator9 : RelationalOperator  Operator===  OutDataTypeStr=boolean  RndMeth=Nearest  InputSameDT=on
  Terminator : Terminator
  TurnOnDelay : CXLib/TurnOnDelay
  TurnOnDelay1 : CXLib/TurnOnDelay
  DFC_RailMeUn3_DSM : Outport  Description=state of DFC_RailMeUn3  OutMin=0  OutMax=1  OutDataTypeStr=boolean
  wires:
  Constant1/1 -> TurnOnDelay1/3
  Constant2/1 -> TurnOnDelay/3
  TurnOnDelay1/1 -> RSFlipFlop/1
  TurnOnDelay/1 -> RSFlipFlop/2
  Constant12/1 -> TurnOnDelay/2
  Logical Operator8/1 -> TurnOnDelay/1
  Constant15/1 -> TurnOnDelay1/2
  Logical Operator6/1 -> TurnOnDelay1/1, Logical Operator8/1  "Rail_stMeUnMon3_mp"
  Logical Operator3/1 -> Logical Operator6/2
  Relational Operator9/1 -> Logical Operator3/1
  Logical Operator5/1 -> Logical Operator3/2
  Rail_stCtlLoop/1 -> Relational Operator9/1
  RailP_pFlt/1 -> Relational Operator8/1
  Epm_nEng/1 -> Rail_pMeUnFltMin_CUR/1
  Rail_pMeUnFltMin_CUR/1 -> Relational Operator8/2  "Rail_pMeUnFltMin_mp"
  Relational Operator8/1 -> Logical Operator6/1
  Constant14/1 -> Relational Operator9/2
  DSM_bRailMeUn3Rls/1 -> Logical Operator9/1
  Logical Operator9/1 -> Logical Operator5/1
  DSM_bRailMeUn3Blk/1 -> Logical Operator5/2
  RSFlipFlop/1 -> DFC_RailMeUn3_DSM/1
  RSFlipFlop/2 -> Terminator/1
  Bitwise Operator/1 -> Compare To Zero/1
  Constant18/1 -> Bitwise Operator/1
  Compare To Zero/1 -> Logical Operator9/2

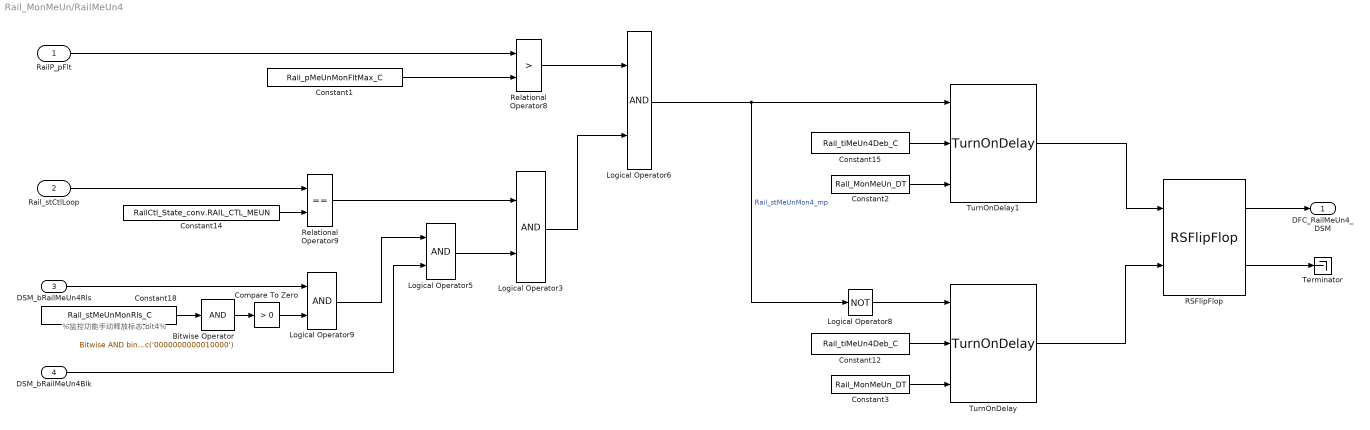
== system Rail_MonMeUn/RailMeUn4 ==
  note: %监控功能手动释放标志,bit4%
  RailP_pFlt : Inport
  Rail_stCtlLoop : Inport  Port=2
  DSM_bRailMeUn4Rls : Inport  Description=state of FId_RailMeUn4Rls  Port=3  OutMin=0  OutMax=1  OutDataTypeStr=boolean
  DSM_bRailMeUn4Blk : Inport  Description=state of FId_RailMeUn4Blk  Port=4  OutMin=0  OutMax=1  OutDataTypeStr=boolean
  Bitwise Operator : simulink/Logic and Bit Operations/Bitwise Operator  logicop=AND  UseBitMask=on  BitMask=bin2dec('0000000000010000')  BitMaskRealWorld=Stored Integer
  Compare To Zero : simulink/Logic and Bit Operations/Compare To Zero  relop=>  OutDataTypeStr=boolean
  Constant1 : Constant  Value=Rail_pMeUnMonFltMax_C
  Constant12 : Constant  Value=Rail_tiMeUn4Deb_C
  Constant14 : Constant  Value=RailCtl_State_conv.RAIL_CTL_MEUN
  Constant15 : Constant  Value=Rail_tiMeUn4Deb_C
  Constant18 : Constant  Value=Rail_stMeUnMonRls_C
  Constant2 : Constant  Value=Rail_MonMeUn_DT  OutDataTypeStr=Inherit: Inherit via back propagation
  Constant3 : Constant  Value=Rail_MonMeUn_DT  OutDataTypeStr=Inherit: Inherit via back propagation
  Logical Operator{3,5..6,9} (4 alike) : Logic  AllPortsSameDT=off  OutDataTypeStr=boolean
  Logical Operator8 : Logic  Operator=NOT  AllPortsSameDT=off  OutDataTypeStr=boolean
  RSFlipFlop : CXLib/RSFlipFlop
  Relational Operator8 : RelationalOperator  Operator=>  OutDataTypeStr=boolean  RndMeth=Nearest  InputSameDT=on
  Relational Operator9 : RelationalOperator  Operator===  OutDataTypeStr=boolean  RndMeth=Nearest  InputSameDT=on
  Terminator : Terminator
  TurnOnDelay : CXLib/TurnOnDelay
  TurnOnDelay1 : CXLib/TurnOnDelay
  DFC_RailMeUn4_DSM : Outport  Description=state of DFC_RailMeUn4  OutMin=0  OutMax=1  OutDataTypeStr=boolean
  wires:
  Constant2/1 -> TurnOnDelay1/3
  Constant3/1 -> TurnOnDelay/3
  TurnOnDelay1/1 -> RSFlipFlop/1
  TurnOnDelay/1 -> RSFlipFlop/2
  Constant12/1 -> TurnOnDelay/2
  Logical Operator8/1 -> TurnOnDelay/1
  Constant15/1 -> TurnOnDelay1/2
  Logical Operator6/1 -> TurnOnDelay1/1, Logical Operator8/1  "Rail_stMeUnMon4_mp"
  Constant1/1 -> Relational Operator8/2
  DSM_bRailMeUn4Blk/1 -> Logical Operator5/2
  Logical Operator9/1 -> Logical Operator5/1
  DSM_bRailMeUn4Rls/1 -> Logical Operator9/1
  Constant14/1 -> Relational Operator9/2
  Relational Operator8/1 -> Logical Operator6/1
  RailP_pFlt/1 -> Relational Operator8/1
  Rail_stCtlLoop/1 -> Relational Operator9/1
  Logical Operator5/1 -> Logical Operator3/2
  Relational Operator9/1 -> Logical Operator3/1
  Logical Operator3/1 -> Logical Operator6/2
  RSFlipFlop/1 -> DFC_RailMeUn4_DSM/1
  RSFlipFlop/2 -> Terminator/1
  Bitwise Operator/1 -> Compare To Zero/1
  Constant18/1 -> Bitwise Operator/1
  Compare To Zero/1 -> Logical Operator9/2

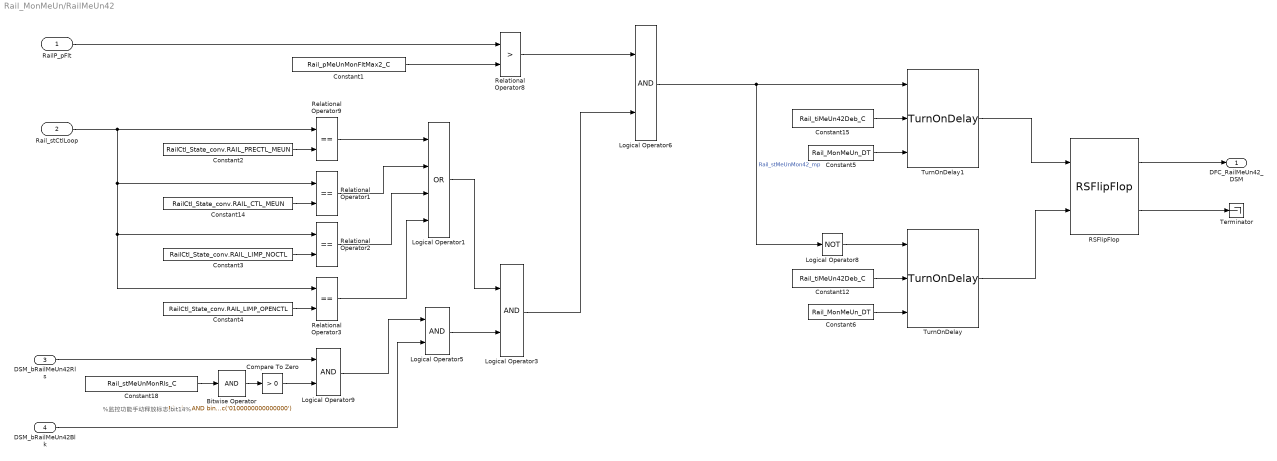
== system Rail_MonMeUn/RailMeUn42 ==
  note: %监控功能手动释放标志,bit14%
  RailP_pFlt : Inport
  Rail_stCtlLoop : Inport  Port=2
  DSM_bRailMeUn42Rls : Inport  Description=state of FId_RailMeUn42Rls  Port=3  OutMin=0  OutMax=1  OutDataTypeStr=boolean
  DSM_bRailMeUn42Blk : Inport  Description=state of FId_RailMeUn42Blk  Port=4  OutMin=0  OutMax=1  OutDataTypeStr=boolean
  Bitwise Operator : simulink/Logic and Bit Operations/Bitwise Operator  logicop=AND  UseBitMask=on  BitMask=bin2dec('0100000000000000')  BitMaskRealWorld=Stored Integer
  Compare To Zero : simulink/Logic and Bit Operations/Compare To Zero  relop=>  OutDataTypeStr=boolean
  Constant1 : Constant  Value=Rail_pMeUnMonFltMax2_C
  Constant12 : Constant  Value=Rail_tiMeUn42Deb_C
  Constant14 : Constant  Value=RailCtl_State_conv.RAIL_CTL_MEUN
  Constant15 : Constant  Value=Rail_tiMeUn42Deb_C
  Constant18 : Constant  Value=Rail_stMeUnMonRls_C
  Constant2 : Constant  Value=RailCtl_State_conv.RAIL_PRECTL_MEUN
  Constant3 : Constant  Value=RailCtl_State_conv.RAIL_LIMP_NOCTL
  Constant4 : Constant  Value=RailCtl_State_conv.RAIL_LIMP_OPENCTL
  Constant5 : Constant  Value=Rail_MonMeUn_DT  OutDataTypeStr=Inherit: Inherit via back propagation
  Constant6 : Constant  Value=Rail_MonMeUn_DT  OutDataTypeStr=Inherit: Inherit via back propagation
  Logical Operator1 : Logic  Operator=OR  Inputs=4  AllPortsSameDT=off  OutDataTypeStr=boolean
  Logical Operator{3,5..6,9} (4 alike) : Logic  AllPortsSameDT=off  OutDataTypeStr=boolean
  Logical Operator8 : Logic  Operator=NOT  AllPortsSameDT=off  OutDataTypeStr=boolean
  RSFlipFlop : CXLib/RSFlipFlop
  Relational Operator{1..3,9} (4 alike) : RelationalOperator  Operator===  OutDataTypeStr=boolean  RndMeth=Nearest  InputSameDT=on
  Relational Operator8 : RelationalOperator  Operator=>  OutDataTypeStr=boolean  RndMeth=Nearest  InputSameDT=on
  Terminator : Terminator
  TurnOnDelay : CXLib/TurnOnDelay
  TurnOnDelay1 : CXLib/TurnOnDelay
  DFC_RailMeUn42_DSM : Outport  Description=state of DFC_RailMeUn42  OutMin=0  OutMax=1  OutDataTypeStr=boolean
  wires:
  Constant5/1 -> TurnOnDelay1/3
  Constant6/1 -> TurnOnDelay/3
  TurnOnDelay1/1 -> RSFlipFlop/1
  TurnOnDelay/1 -> RSFlipFlop/2
  Constant12/1 -> TurnOnDelay/2
  Logical Operator8/1 -> TurnOnDelay/1
  Constant15/1 -> TurnOnDelay1/2
  Logical Operator6/1 -> TurnOnDelay1/1, Logical Operator8/1  "Rail_stMeUnMon42_mp"
  Relational Operator8/1 -> Logical Operator6/1
  Logical Operator3/1 -> Logical Operator6/2
  Logical Operator1/1 -> Logical Operator3/1
  Constant3/1 -> Relational Operator2/2
  Constant4/1 -> Relational Operator3/2
  Relational Operator3/1 -> Logical Operator1/4
  Relational Operator2/1 -> Logical Operator1/3
  Constant14/1 -> Relational Operator1/2
  Relational Operator1/1 -> Logical Operator1/2
  Relational Operator9/1 -> Logical Operator1/1
  Logical Operator5/1 -> Logical Operator3/2
  Rail_stCtlLoop/1 -> Relational Operator9/1, Relational Operator1/1, Relational Operator2/1, Relational Operator3/1
  RailP_pFlt/1 -> Relational Operator8/1
  Constant2/1 -> Relational Operator9/2
  DSM_bRailMeUn42Rls/1 -> Logical Operator9/1
  Logical Operator9/1 -> Logical Operator5/1
  DSM_bRailMeUn42Blk/1 -> Logical Operator5/2
  Constant1/1 -> Relational Operator8/2
  RSFlipFlop/1 -> DFC_RailMeUn42_DSM/1
  RSFlipFlop/2 -> Terminator/1
  Bitwise Operator/1 -> Compare To Zero/1
  Constant18/1 -> Bitwise Operator/1
  Compare To Zero/1 -> Logical Operator9/2

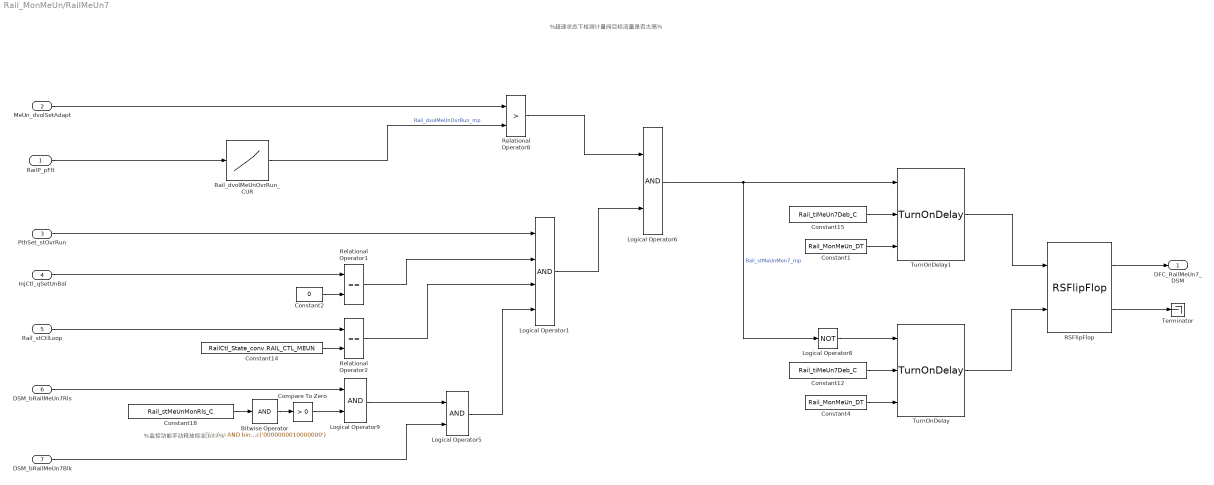
== system Rail_MonMeUn/RailMeUn7 ==
  note: %超速状态下检测计量阀目标流量是否太高%
  note: %监控功能手动释放标志,bit7%
  RailP_pFlt : Inport
  MeUn_dvolSetAdapt : Inport  Port=2
  PthSet_stOvrRun : Inport  Port=3
  InjCtl_qSetUnBal : Inport  Port=4
  Rail_stCtlLoop : Inport  Port=5
  DSM_bRailMeUn7Rls : Inport  Description=state of FId_RailMeUn7Rls  Port=6  OutMin=0  OutMax=1  OutDataTypeStr=boolean
  DSM_bRailMeUn7Blk : Inport  Description=state of FId_RailMeUn7Blk  Port=7  OutMin=0  OutMax=1  OutDataTypeStr=boolean
  Bitwise Operator : simulink/Logic and Bit Operations/Bitwise Operator  logicop=AND  UseBitMask=on  BitMask=bin2dec('0000000010000000')  BitMaskRealWorld=Stored Integer
  Compare To Zero : simulink/Logic and Bit Operations/Compare To Zero  relop=>  OutDataTypeStr=boolean
  Constant1 : Constant  Value=Rail_MonMeUn_DT  OutDataTypeStr=Inherit: Inherit via back propagation
  Constant12 : Constant  Value=Rail_tiMeUn7Deb_C
  Constant14 : Constant  Value=RailCtl_State_conv.RAIL_CTL_MEUN
  Constant15 : Constant  Value=Rail_tiMeUn7Deb_C
  Constant18 : Constant  Value=Rail_stMeUnMonRls_C
  Constant2 : Constant  Value=0  OutDataTypeStr=Inherit: Inherit via back propagation
  Constant4 : Constant  Value=Rail_MonMeUn_DT  OutDataTypeStr=Inherit: Inherit via back propagation
  Logical Operator1 : Logic  Inputs=4  AllPortsSameDT=off  OutDataTypeStr=boolean
  Logical Operator5 : Logic  AllPortsSameDT=off  OutDataTypeStr=boolean
  Logical Operator6 : Logic  AllPortsSameDT=off  OutDataTypeStr=boolean
  Logical Operator8 : Logic  Operator=NOT  AllPortsSameDT=off  OutDataTypeStr=boolean
  Logical Operator9 : Logic  AllPortsSameDT=off  OutDataTypeStr=boolean
  RSFlipFlop : CXLib/RSFlipFlop
  Rail_dvolMeUnOvrRun_CUR : Lookup_n-D  NumberOfTableDimensions=1  BreakpointsForDimension1=Rail_dvolMeUnOvrRun_CURX  IndexSearchMethod=Linear search  Table=Rail_dvolMeUnOvrRun_CUR  ExtrapMethod=Clip  InternalRulePriority=Speed  OutDataTypeStr=Inherit: Inherit via back propagation  RndMeth=Simplest  SaturateOnIntegerOverflow=on
  Relational Operator1 : RelationalOperator  Operator===  OutDataTypeStr=boolean  RndMeth=Nearest  InputSameDT=on
  Relational Operator2 : RelationalOperator  Operator===  OutDataTypeStr=boolean  RndMeth=Nearest  InputSameDT=on
  Relational Operator8 : RelationalOperator  Operator=>  OutDataTypeStr=boolean  RndMeth=Nearest  InputSameDT=on
  Terminator : Terminator
  TurnOnDelay : CXLib/TurnOnDelay
  TurnOnDelay1 : CXLib/TurnOnDelay
  DFC_RailMeUn7_DSM : Outport  Description=state of DFC_RailMeUn7  OutMin=0  OutMax=1  OutDataTypeStr=boolean
  wires:
  Constant1/1 -> TurnOnDelay1/3
  Constant4/1 -> TurnOnDelay/3
  TurnOnDelay1/1 -> RSFlipFlop/1
  TurnOnDelay/1 -> RSFlipFlop/2
  Constant12/1 -> TurnOnDelay/2
  Logical Operator8/1 -> TurnOnDelay/1
  Constant15/1 -> TurnOnDelay1/2
  Logical Operator6/1 -> TurnOnDelay1/1, Logical Operator8/1  "Rail_stMeUnMon7_mp"
  Logical Operator5/1 -> Logical Operator1/4
  Rail_stCtlLoop/1 -> Relational Operator2/1
  InjCtl_qSetUnBal/1 -> Relational Operator1/1
  PthSet_stOvrRun/1 -> Logical Operator1/1
  Logical Operator1/1 -> Logical Operator6/2
  MeUn_dvolSetAdapt/1 -> Relational Operator8/1
  RailP_pFlt/1 -> Rail_dvolMeUnOvrRun_CUR/1
  Rail_dvolMeUnOvrRun_CUR/1 -> Relational Operator8/2  "Rail_dvolMeUnOvrRun_mp"
  DSM_bRailMeUn7Blk/1 -> Logical Operator5/2
  Logical Operator9/1 -> Logical Operator5/1
  DSM_bRailMeUn7Rls/1 -> Logical Operator9/1
  Relational Operator8/1 -> Logical Operator6/1
  Relational Operator1/1 -> Logical Operator1/2
  Constant2/1 -> Relational Operator1/2
  Relational Operator2/1 -> Logical Operator1/3
  Constant14/1 -> Relational Operator2/2
  RSFlipFlop/1 -> DFC_RailMeUn7_DSM/1
  RSFlipFlop/2 -> Terminator/1
  Bitwise Operator/1 -> Compare To Zero/1
  Constant18/1 -> Bitwise Operator/1
  Compare To Zero/1 -> Logical Operator9/2

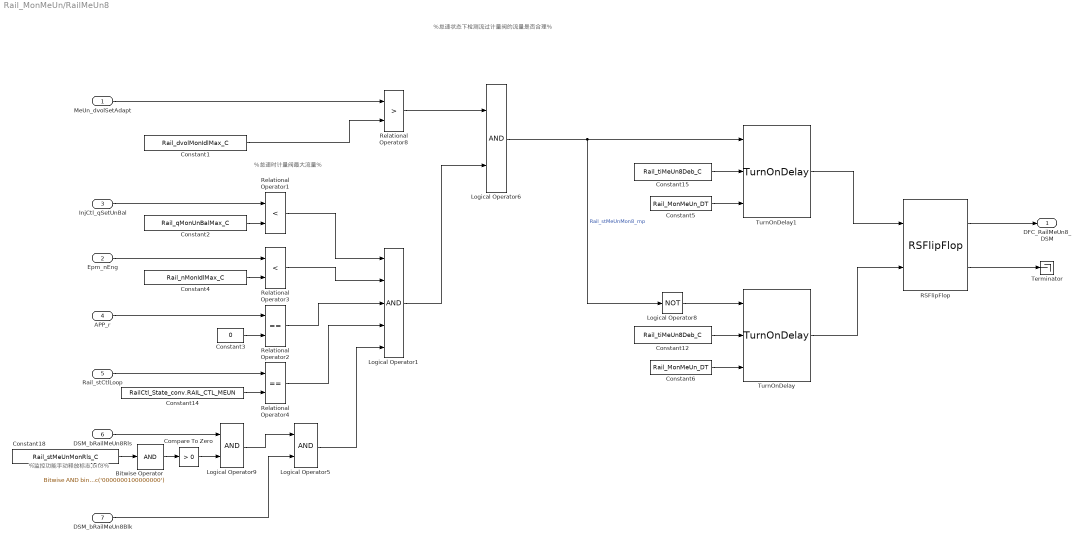
== system Rail_MonMeUn/RailMeUn8 ==
  note: %怠速状态下检测流过计量阀的流量是否合理%
  note: %怠速时计量阀最大流量%
  note: %监控功能手动释放标志,bit8%
  MeUn_dvolSetAdapt : Inport
  Epm_nEng : Inport  Port=2
  InjCtl_qSetUnBal : Inport  Port=3
  APP_r : Inport  Port=4
  Rail_stCtlLoop : Inport  Port=5
  DSM_bRailMeUn8Rls : Inport  Description=state of FId_RailMeUn8Rls  Port=6  OutMin=0  OutMax=1  OutDataTypeStr=boolean
  DSM_bRailMeUn8Blk : Inport  Description=state of FId_RailMeUn8Blk  Port=7  OutMin=0  OutMax=1  OutDataTypeStr=boolean
  Bitwise Operator : simulink/Logic and Bit Operations/Bitwise Operator  logicop=AND  UseBitMask=on  BitMask=bin2dec('0000000100000000')  BitMaskRealWorld=Stored Integer
  Compare To Zero : simulink/Logic and Bit Operations/Compare To Zero  relop=>  OutDataTypeStr=boolean
  Constant1 : Constant  Value=Rail_dvolMonIdlMax_C
  Constant12 : Constant  Value=Rail_tiMeUn8Deb_C
  Constant14 : Constant  Value=RailCtl_State_conv.RAIL_CTL_MEUN
  Constant15 : Constant  Value=Rail_tiMeUn8Deb_C
  Constant18 : Constant  Value=Rail_stMeUnMonRls_C
  Constant2 : Constant  Value=Rail_qMonUnBalMax_C
  Constant3 : Constant  Value=0  OutDataTypeStr=Inherit: Inherit via back propagation
  Constant4 : Constant  Value=Rail_nMonIdlMax_C
  Constant5 : Constant  Value=Rail_MonMeUn_DT  OutDataTypeStr=Inherit: Inherit via back propagation
  Constant6 : Constant  Value=Rail_MonMeUn_DT  OutDataTypeStr=Inherit: Inherit via back propagation
  Logical Operator1 : Logic  Inputs=5  AllPortsSameDT=off  OutDataTypeStr=boolean
  Logical Operator5 : Logic  AllPortsSameDT=off  OutDataTypeStr=boolean
  Logical Operator6 : Logic  AllPortsSameDT=off  OutDataTypeStr=boolean
  Logical Operator8 : Logic  Operator=NOT  AllPortsSameDT=off  OutDataTypeStr=boolean
  Logical Operator9 : Logic  AllPortsSameDT=off  OutDataTypeStr=boolean
  RSFlipFlop : CXLib/RSFlipFlop
  Relational Operator1 : RelationalOperator  Operator=<  OutDataTypeStr=boolean  RndMeth=Nearest  InputSameDT=on
  Relational Operator2 : RelationalOperator  Operator===  OutDataTypeStr=boolean  RndMeth=Nearest  InputSameDT=on
  Relational Operator3 : RelationalOperator  Operator=<  OutDataTypeStr=boolean  RndMeth=Nearest  InputSameDT=on
  Relational Operator4 : RelationalOperator  Operator===  OutDataTypeStr=boolean  RndMeth=Nearest  InputSameDT=on
  Relational Operator8 : RelationalOperator  Operator=>  OutDataTypeStr=boolean  RndMeth=Nearest  InputSameDT=on
  Terminator : Terminator
  TurnOnDelay : CXLib/TurnOnDelay
  TurnOnDelay1 : CXLib/TurnOnDelay
  DFC_RailMeUn8_DSM : Outport  Description=state of DFC_RailMeUn8  OutMin=0  OutMax=1  OutDataTypeStr=boolean
  wires:
  Constant5/1 -> TurnOnDelay1/3
  Constant6/1 -> TurnOnDelay/3
  Logical Operator8/1 -> TurnOnDelay/1
  TurnOnDelay1/1 -> RSFlipFlop/1
  TurnOnDelay/1 -> RSFlipFlop/2
  Constant12/1 -> TurnOnDelay/2
  Constant15/1 -> TurnOnDelay1/2
  Logical Operator6/1 -> TurnOnDelay1/1, Logical Operator8/1  "Rail_stMeUnMon8_mp"
  Logical Operator5/1 -> Logical Operator1/5
  Relational Operator4/1 -> Logical Operator1/4
  Rail_stCtlLoop/1 -> Relational Operator4/1
  Constant14/1 -> Relational Operator4/2
  Relational Operator2/1 -> Logical Operator1/3
  Relational Operator3/1 -> Logical Operator1/2
  Constant4/1 -> Relational Operator3/2
  Epm_nEng/1 -> Relational Operator3/1
  Relational Operator1/1 -> Logical Operator1/1
  Constant2/1 -> Relational Operator1/2
  Constant1/1 -> Relational Operator8/2
  Constant3/1 -> Relational Operator2/2
  Relational Operator8/1 -> Logical Operator6/1
  DSM_bRailMeUn8Rls/1 -> Logical Operator9/1
  Logical Operator9/1 -> Logical Operator5/1
  DSM_bRailMeUn8Blk/1 -> Logical Operator5/2
  MeUn_dvolSetAdapt/1 -> Relational Operator8/1
  Logical Operator1/1 -> Logical Operator6/2
  InjCtl_qSetUnBal/1 -> Relational Operator1/1
  APP_r/1 -> Relational Operator2/1
  RSFlipFlop/1 -> DFC_RailMeUn8_DSM/1
  RSFlipFlop/2 -> Terminator/1
  Bitwise Operator/1 -> Compare To Zero/1
  Constant18/1 -> Bitwise Operator/1
  Compare To Zero/1 -> Logical Operator9/2
